simulink model "test_Tustin"  (R2023a)
settings: Solver=VariableStepAuto  StartTime=0.0  StopTime=30  RelTol=1e-3
InitFcn:
  | clear mex
values from neighbouring files (symbols this model uses):
  Gp = K / (tau*s+1)    [controller.m]
undefined symbols (not defined in the file or in its folder): den, Grd1, Grd2, num
settings Model: Creator=Sandor  LastModifiedBy=Enio
settings DebuggingCC: UnconnectedInputMsg=warning  UnconnectedOutputMsg=warning  UnconnectedLineMsg=warning
settings ModelReferenceCC: EnableRefExpFcnMdlSchedulingChecks=on
settings SFSimCC: SimCustomHeaderCode="#include \"controller.h\""  SimUserSources=controller.c
settings RTWCC: DLArmComputeVersion=19.05

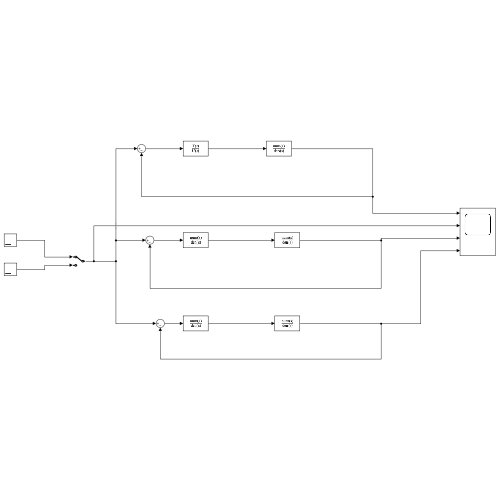
[thumbnail: Simulink's stored preview of the top-level diagram]
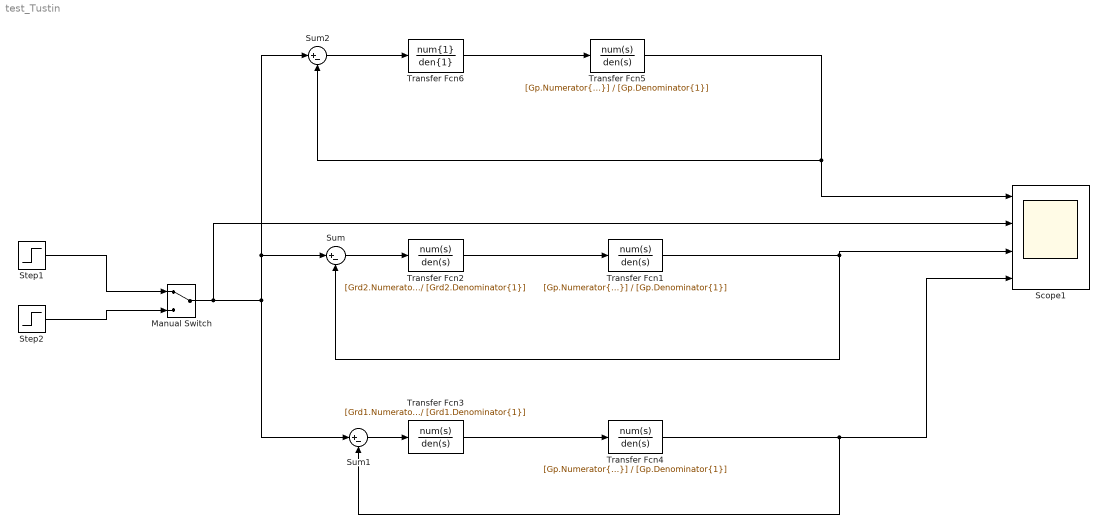
== system test_Tustin ==
  Manual Switch : ManualSwitch
  Scope1 : Scope  NumInputPorts=4
  Step1 : Step  Time=0  After=6  SampleTime=0
  Step2 : Step  Time=0  After=60  SampleTime=0
  Sum : Sum  Inputs=|+-
  Sum1 : Sum  Inputs=|+-
  Sum2 : Sum  Inputs=|+-
  Transfer Fcn1 : TransferFcn  Numerator=[Gp.Numerator{1}]  Denominator=[Gp.Denominator{1}]
  Transfer Fcn2 : TransferFcn  Numerator=[Grd2.Numerator{1}]  Denominator=[Grd2.Denominator{1}]
  Transfer Fcn3 : TransferFcn  Numerator=[Grd1.Numerator{1}]  Denominator=[Grd1.Denominator{1}]
  Transfer Fcn4 : TransferFcn  Numerator=[Gp.Numerator{1}]  Denominator=[Gp.Denominator{1}]
  Transfer Fcn5 : TransferFcn  Numerator=[Gp.Numerator{1}]  Denominator=[Gp.Denominator{1}]
  Transfer Fcn6 : TransferFcn  Numerator=num{1}  Denominator=den{1}
  wires:
  Transfer Fcn3/1 -> Transfer Fcn4/1
  Transfer Fcn1/1 -> Sum/2, Scope1/3
  Step1/1 -> Manual Switch/1
  Transfer Fcn4/1 -> Sum1/2, Scope1/4
  Sum1/1 -> Transfer Fcn3/1
  Transfer Fcn2/1 -> Transfer Fcn1/1
  Sum/1 -> Transfer Fcn2/1
  Step2/1 -> Manual Switch/2
  Manual Switch/1 -> Scope1/2, Sum2/1, Sum/1, Sum1/1
  Transfer Fcn5/1 -> Scope1/1, Sum2/2
  Transfer Fcn6/1 -> Transfer Fcn5/1
  Sum2/1 -> Transfer Fcn6/1
